simulink model "piControllerLoad"  (R2024a)
settings: Solver=VariableStepAuto  StartTime=0.0  StopTime=20  RelTol=1e-3
settings Model: Creator=janho  LastModifiedBy=janho

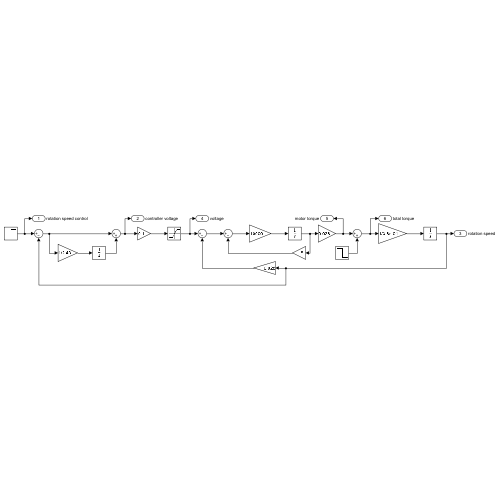
[thumbnail: Simulink's stored preview of the top-level diagram]
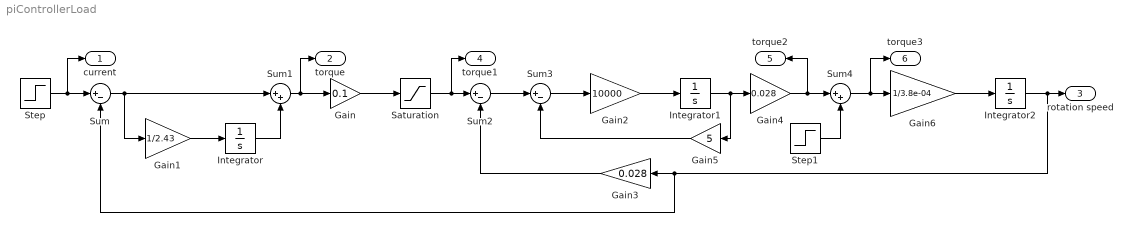
== system piControllerLoad ==
  Gain : Gain  Gain=0.1
  Gain1 : Gain  Gain=1/2.43
  Gain2 : Gain  Gain=10000
  Gain3 : Gain  Gain=0.028
  Gain4 : Gain  Gain=0.028
  Gain5 : Gain  Gain=5
  Gain6 : Gain  Gain=1/3.8e-04
  Integrator : Integrator
  Integrator1 : Integrator
  Integrator2 : Integrator
  Saturation : Saturate  UpperLimit=10  LowerLimit=-10
  Step : Step  Time=0  After=100  SampleTime=0
  Step1 : Step  Time=10  After=-0.01  SampleTime=0
  Sum : Sum  Inputs=|+-
  Sum1 : Sum  Inputs=|++
  Sum2 : Sum  Inputs=|+-
  Sum3 : Sum  Inputs=|+-
  Sum4 : Sum  Inputs=|++
  current : Outport  SignalName=rotation speed control
  torque : Outport  Port=2  SignalName=controller voltage
  rotation speed : Outport  Port=3  SignalName=rotation speed
  torque1 : Outport  Port=4  SignalName=voltage
  torque2 : Outport  Port=5  SignalName=motor torque
  torque3 : Outport  Port=6  SignalName=total torque
  wires:
  Sum/1 -> Sum1/1, Gain1/1
  Step/1 -> current/1, Sum/1
  Sum1/1 -> torque/1, Gain/1
  Gain/1 -> Saturation/1
  Integrator/1 -> Sum1/2
  Gain1/1 -> Integrator/1
  Sum3/1 -> Gain2/1
  Sum2/1 -> Sum3/1
  Saturation/1 -> torque1/1, Sum2/1
  Gain3/1 -> Sum2/2
  Gain5/1 -> Sum3/2
  Integrator2/1 -> rotation speed/1, Gain3/1, Sum/2
  Integrator1/1 -> Gain4/1, Gain5/1
  Gain2/1 -> Integrator1/1
  Gain6/1 -> Integrator2/1
  Gain4/1 -> Sum4/1, torque2/1
  Sum4/1 -> Gain6/1, torque3/1
  Step1/1 -> Sum4/2
